simulink model "ft_modelo"  (R2023a)
settings: Solver=FixedStepAuto  StartTime=0.0  StopTime=3.26  FixedStep=1e-4  RelTol=1e-3
model workspace (MAT data in the model file):
  B = 0.00071
  J = 0.0021
  Ke = 0.0921
  Kt = 0.0921
  L = 0.000228912
  R = 2.8614
values from neighbouring files (symbols this model uses):
  Ta = L/R    (= 8e-05)    [ft_motor.m]
  Tb = J/b    (= 3)    [ft_motor.m]
  Tm = R*J/(Ke*Kt)    (= 0.718520090399)    [ft_motor.m]
libraries: simulink x1
settings Model: Creator=Alexandre  LastModifiedBy=Alexandre
settings SolverCC: AlgebraicLoopSolver=TrustRegion

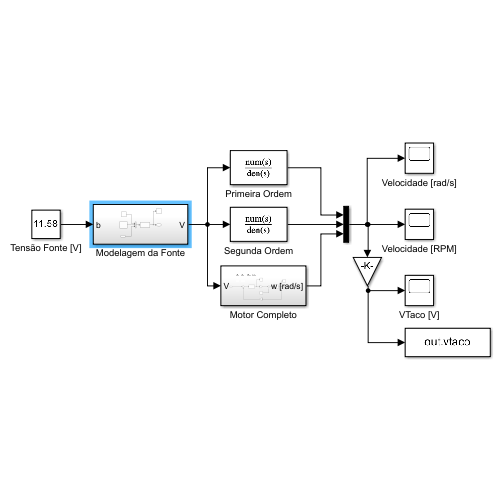
[thumbnail: Simulink's stored preview of the top-level diagram]
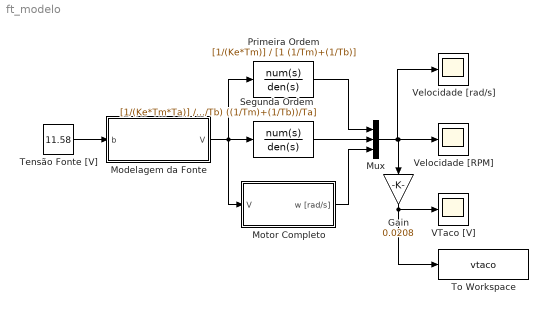
== system ft_modelo ==
  Gain : Gain  Gain=0.0208
  Modelagem da Fonte : Subsystem
  Motor Completo : Subsystem
  Mux : Mux  Inputs=3
  Primeira Ordem : TransferFcn  Numerator=[1/(Ke*Tm)]  Denominator=[1 (1/Tm)+(1/Tb)]
  Segunda Ordem : TransferFcn  Numerator=[1/(Ke*Tm*Ta)]  Denominator=[1 (1/Tm)+(1/Tb) ((1/Tm)+(1/Tb))/Ta]
  Tensão Fonte [V] : Constant  Value=11.58
  To Workspace : ToWorkspace  VariableName=vtaco  SaveFormat=Timeseries  SampleTime=-1
  VTaco [V] : Scope
  Velocidade [RPM] : Scope
  Velocidade [rad/s] : Scope
  wires:
  Modelagem da Fonte/1(V) -> Segunda Ordem/1, Primeira Ordem/1, Motor Completo/1(V)
  Mux/1 -> Gain/1, Velocidade [RPM]/1, Velocidade [rad/s]/1
  Primeira Ordem/1 -> Mux/1
  Segunda Ordem/1 -> Mux/2
  Tensão Fonte [V]/1 -> Modelagem da Fonte/1(b)
  Gain/1 -> To Workspace/1, VTaco [V]/1
  Motor Completo/1(w [rad/s]) -> Mux/3

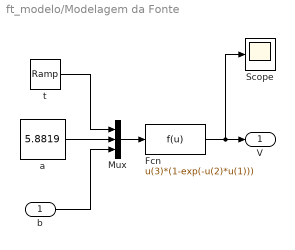
== system ft_modelo/Modelagem da Fonte ==
  b : Inport
  Fcn : Fcn  Expr=u(3)*(1-exp(-u(2)*u(1)))
  Mux : Mux  Inputs=3
  Scope : Scope
  a : Constant  Value=5.8819
  t : simulink/Sources/Ramp  slope=1  start=0  InitialOutput=0
  V : Outport
  wires:
  Mux/1 -> Fcn/1
  t/1 -> Mux/1
  Fcn/1 -> V/1, Scope/1
  a/1 -> Mux/2
  b/1 -> Mux/3

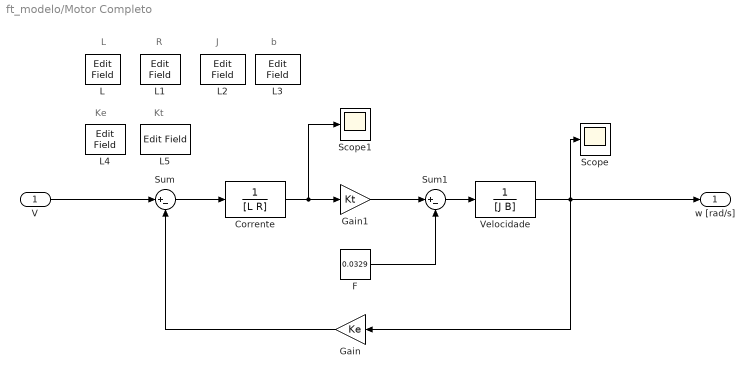
== system ft_modelo/Motor Completo ==
  note: Ke
  note: R
  note: b
  note: J
  note: Kt
  note: L
  V : Inport
  Corrente : TransferFcn  Denominator=[L R]
  F : Constant  Value=0.0329
  Gain : Gain  Gain=Ke
  Gain1 : Gain  Gain=Kt
  L{,1..5} (6 alike) : EditField  LabelPosition=Hide  ShowInitialText=on  Alignment=Center
  Scope : Scope
  Scope1 : Scope
  Sum : Sum  Inputs=|+-
  Sum1 : Sum  Inputs=|+-
  Velocidade : TransferFcn  Denominator=[J B]
  w [rad/s] : Outport
  wires:
  Gain/1 -> Sum/2
  Sum/1 -> Corrente/1
  Sum1/1 -> Velocidade/1
  Gain1/1 -> Sum1/1
  F/1 -> Sum1/2
  Velocidade/1 -> w [rad/s]/1, Scope/1, Gain/1
  Corrente/1 -> Scope1/1, Gain1/1
  V/1 -> Sum/1
